simulink model "class5_quiz_sumulik1_solution"  (R2019b)
settings: Solver=VariableStepAuto  StartTime=0.0  StopTime=10.0  RelTol=1e-3
settings Model: Creator=Rashedul Islam  LastModifiedBy=Rashedul Islam

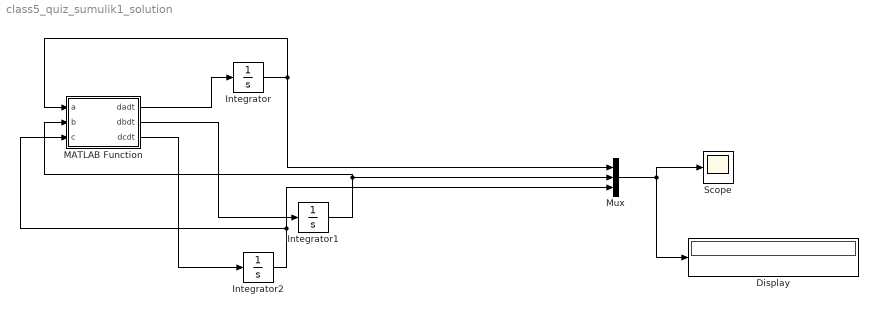
== system class5_quiz_sumulik1_solution ==
  Display : Display
  Integrator : Integrator  InitialCondition=100
  Integrator1 : Integrator  InitialCondition=200
  Integrator2 : Integrator
  MATLAB Function : MATLAB Function  TreatAsAtomicUnit=on
  Mux : Mux  Inputs=3
  Scope : Scope
  wires:
  MATLAB Function/1(dadt) -> Integrator/1
  Integrator/1 -> Mux/1, MATLAB Function/1(a)
  MATLAB Function/2(dbdt) -> Integrator1/1
  Integrator1/1 -> Mux/2, MATLAB Function/2(b)
  MATLAB Function/3(dcdt) -> Integrator2/1
  Integrator2/1 -> Mux/3, MATLAB Function/3(c)
  Mux/1 -> Display/1, Scope/1

== matlab function class5_quiz_sumulik1_solution/MATLAB Function ==
  data: a input; b input; c input; dadt output; dbdt output; dcdt output
function [dadt,dbdt,dcdt] = fcn(a,b,c)
k1=.001;
k2=.1;
%c=0;
%b=200;
%a+b==2*c;
dadt=(k2*c)-k1*a*b ;
dbdt=(k2*c)-k1*a*b ;
dcdt=(2*k1*a*b)-(2*k2*c);
